simulink model "Copy_of_B747"  (R2022b)
settings: Solver=VariableStepAuto  StartTime=0.0  StopTime=Inf  RelTol=1e-3
undefined symbols (not defined in the file): Initial_cond, Interpolation, out_tr
libraries: simulink_extras x9, slpidlib x5, simulink x3, aerolibanimutils x1
settings Model: Creator=Usuario  LastModifiedBy=Usuario

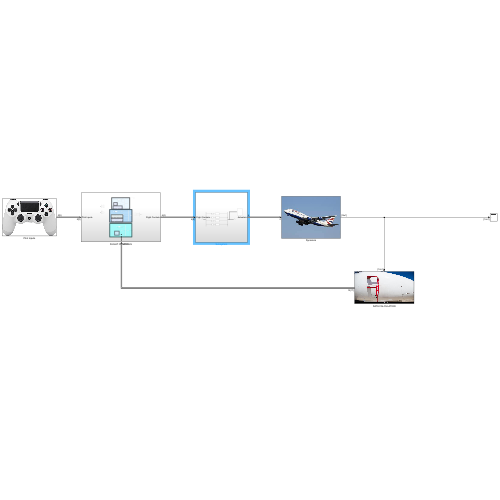
[thumbnail: Simulink's stored preview of the top-level diagram]
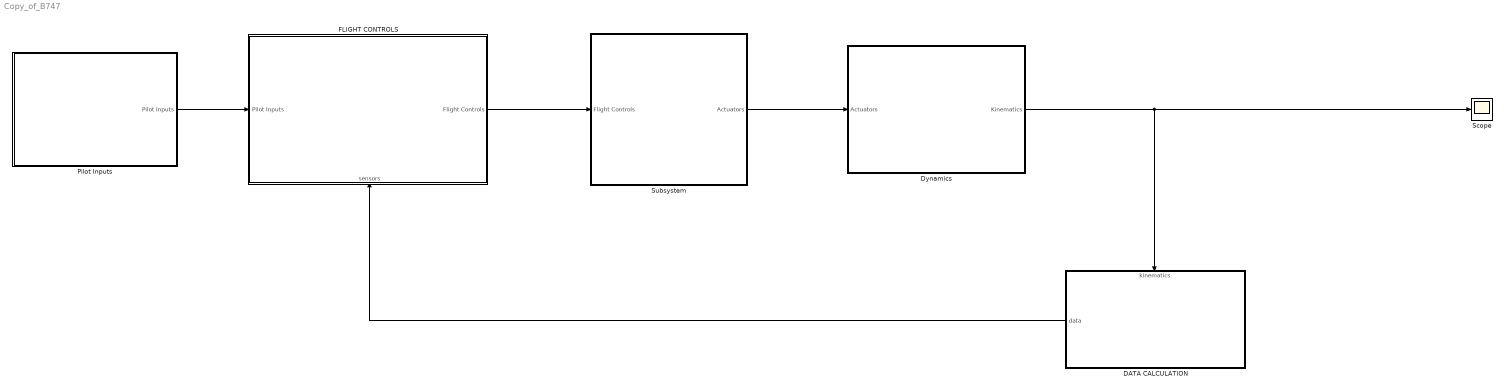
== system Copy_of_B747 ==
  DATA CALCULATION : Subsystem
      settings: PortSchema="{\"entries\":[{\"content\":{\"sides\":[{\"content\":{\"connectorIds\":[\"Out1\"]},\"type\":\"ConnectorPlacement.EquallySpacedRectSide\",\"uuid\":\"3684fda8-23e5-43c4-a1a0-31248e0867f7\"},{\"content\":{\"connectorIds\":[],\"side\":\"RIGHT\"},\"type\":\"ConnectorPlacement.EquallySpacedRectSide\",\"uuid\":\"596d4b37-a63d-424d-8484-dfaf2b397c2c\"},{\"content\":{\"connectorIds\":[\"In1\"],\"side\":\"TOP\"},\"type\":\"ConnectorPlacement.EquallySpacedRectSide\",\"uuid\":\"a12e15c3-f725-45e6-985f-961936170549\"}]},\"type\":\"ConnectorPlacement.EquallySpacedConnector\",\"uuid\":\"9a86d170-49a6-41d6-b658-373aeeb8993b\"}],\"packageUris\":[\"http://schema.mathworks.com/mf0/Connector/R2020b\"],\"version\":\"1.0\"}"
      mask Display: image('C:\Users\Usuario\Documents\MATLAB\B737_simulator\TFM_pics\tubo pitot.jpg'); % Use "Edit Image" on toolstrip to change.
  Dynamics : Subsystem
      mask Display: image('C:\Users\Usuario\Documents\MATLAB\B737_simulator\TFM_pics\b747.jpg'); % Use "Edit Image" on toolstrip to change.
  FLIGHT CONTROLS : Subsystem
      settings: PortSchema="{\"entries\":[{\"content\":{\"sides\":[{\"content\":{\"connectorIds\":[\"In1\"]},\"type\":\"ConnectorPlacement.EquallySpacedRectSide\",\"uuid\":\"91b83ee8-c6ec-4ad7-b4f3-f14dc1cf5d1a\"},{\"content\":{\"connectorIds\":[\"Out1\"],\"side\":\"RIGHT\"},\"type\":\"ConnectorPlacement.EquallySpacedRectSide\",\"uuid\":\"e219be01-4a6e-4062-b72b-ec1396091ca7\"},{\"content\":{\"connectorIds\":[],\"side\":\"TOP\"},\"type\":\"ConnectorPlacement.EquallySpacedRectSide\",\"uuid\":\"96cbe711-5ed8-4304-ab27-a44b299b9c71\"},{\"content\":{\"connectorIds\":[\"In2\"],\"side\":\"BOTTOM\"},\"type\":\"ConnectorPlacement.EquallySpacedRectSide\",\"uuid\":\"b42a0dac-2e5b-48eb-828b-7619874c0cc5\"}]},\"type\":\"ConnectorPlacement.EquallySpacedConnector\",\"uuid\":\"6f7a40d1-3b47-47bb-8706-2539ab3d82b8\"}],\"packageUris\":[\"http://schema.mathworks.com/mf0/Connector/R2020b\"],\"version\":\"1.0\"}"
  Pilot Inputs : Subsystem
      mask Display: image('C:\Users\Usuario\Desktop\mando.jpg'); % Use "Edit Image" on toolstrip to change.
  Scope : Scope
  Subsystem : Subsystem
  wires:
  Dynamics/1(Kinematics) -> Scope/1, DATA CALCULATION/1(kinematics)
  FLIGHT CONTROLS/1(Flight Controls) -> Subsystem/1(Flight Controls)
  DATA CALCULATION/1(data) -> FLIGHT CONTROLS/2(sensors)
  Pilot Inputs/1(Pilot Inputs) -> FLIGHT CONTROLS/1(Pilot Inputs)
  Subsystem/1(Actuators) -> Dynamics/1(Actuators)

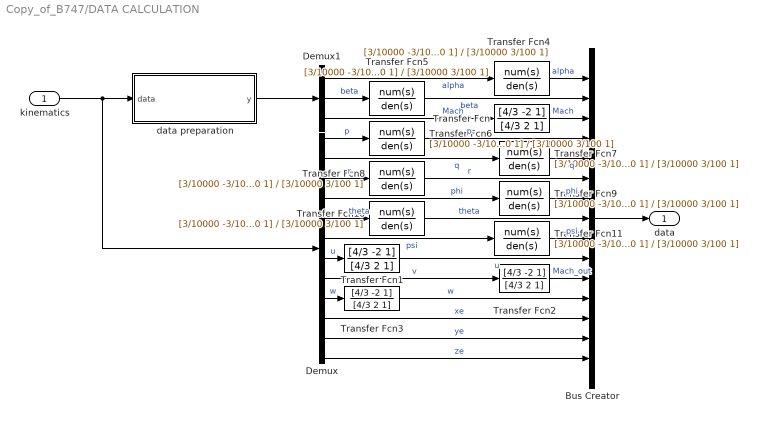
== system Copy_of_B747/DATA CALCULATION ==
  kinematics : Inport
  Bus Creator : BusCreator  Inputs=15
  Demux : Demux  Outputs=12
  Demux1 : Demux  Outputs=3
  Transfer Fcn{,1..3} (4 alike) : TransferFcn  Numerator=[4/3 -2 1]  Denominator=[4/3 2 1]
  Transfer Fcn{4..11} (8 alike) : TransferFcn  Numerator=[3/10000 -3/100 1]  Denominator=[3/10000 3/100 1]
  data preparation : MATLAB Function  TreatAsAtomicUnit=on
  data : Outport
  wires:
  kinematics/1 -> data preparation/1(data), Demux/1
  data preparation/1(y) -> Demux1/1
  Demux1/1 -> Transfer Fcn4/1  "alpha"
  Demux1/2 -> Transfer Fcn5/1  "beta"
  Demux1/3 -> Transfer Fcn/1  "Mach"
  Demux/1 -> Transfer Fcn6/1  "p"
  Demux/2 -> Transfer Fcn7/1  "q"
  Demux/3 -> Transfer Fcn8/1  "r"
  Demux/4 -> Transfer Fcn9/1  "phi"
  Demux/5 -> Transfer Fcn10/1  "theta"
  Demux/6 -> Transfer Fcn11/1  "psi"
  Demux/7 -> Transfer Fcn1/1  "u"
  Demux/8 -> Transfer Fcn2/1  "v"
  Demux/9 -> Transfer Fcn3/1  "w"
  Demux/10 -> Bus Creator/13  "xe"
  Demux/11 -> Bus Creator/14  "ye"
  Demux/12 -> Bus Creator/15  "ze"
  Bus Creator/1 -> data/1
  Transfer Fcn/1 -> Bus Creator/3  "Mach"
  Transfer Fcn1/1 -> Bus Creator/10  "u"
  Transfer Fcn2/1 -> Bus Creator/11  "Mach_out"
  Transfer Fcn3/1 -> Bus Creator/12  "w"
  Transfer Fcn4/1 -> Bus Creator/1  "alpha"
  Transfer Fcn5/1 -> Bus Creator/2  "beta"
  Transfer Fcn6/1 -> Bus Creator/4  "p"
  Transfer Fcn7/1 -> Bus Creator/5  "q"
  Transfer Fcn8/1 -> Bus Creator/6  "r"
  Transfer Fcn9/1 -> Bus Creator/7  "phi"
  Transfer Fcn10/1 -> Bus Creator/8  "theta"
  Transfer Fcn11/1 -> Bus Creator/9  "psi"

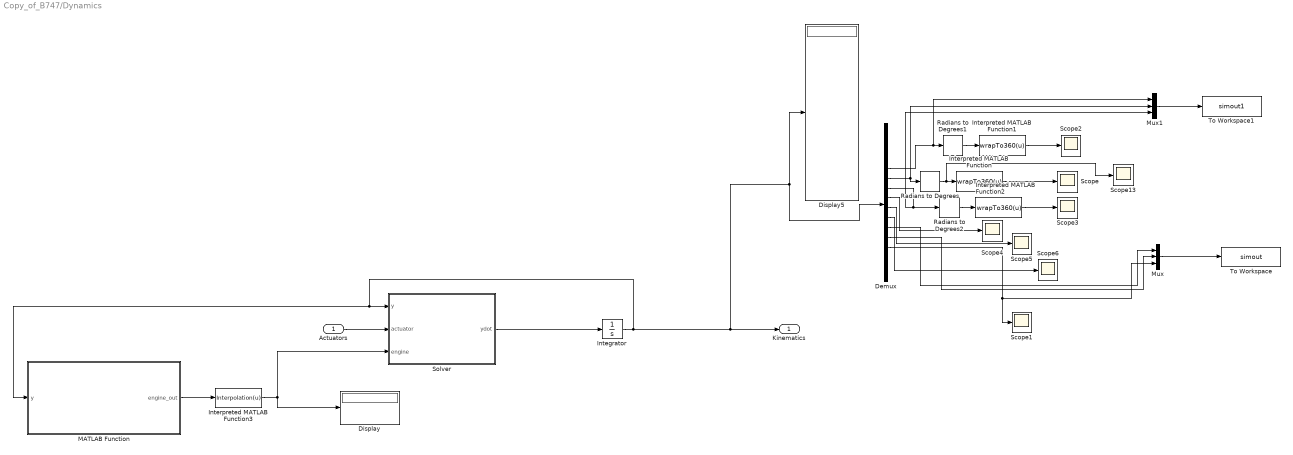
== system Copy_of_B747/Dynamics ==
  Actuators : Inport
  Demux : Demux  Outputs=14
  Display : Display
  Display5 : Display
  Integrator : Integrator  InitialCondition=Initial_cond  ContinuousStateAttributes={'p','q','r','phi','theta','psi','u','v','w','x','y','z','lat','lon'}
  Interpreted MATLAB Function : MATLABFcn  MATLABFcn=wrapTo360(u)
  Interpreted MATLAB Function1 : MATLABFcn  MATLABFcn=wrapTo360(u)
  Interpreted MATLAB Function2 : MATLABFcn  MATLABFcn=wrapTo360(u)
  Interpreted MATLAB Function3 : MATLABFcn  MATLABFcn=Interpolation(u)
  MATLAB Function : MATLAB Function  TreatAsAtomicUnit=on
  Mux : Mux  Inputs=3
  Mux1 : Mux  Inputs=3
  Radians to Degrees : simulink_extras/Transformations/Radians to Degrees
  Radians to Degrees1 : simulink_extras/Transformations/Radians to Degrees
  Radians to Degrees2 : simulink_extras/Transformations/Radians to Degrees
  Scope{,1..6,13} (8 alike) : Scope
  Solver : MATLAB Function  TreatAsAtomicUnit=on
  To Workspace : ToWorkspace  VariableName=simout  SampleTime=-1
  To Workspace1 : ToWorkspace  VariableName=simout1  SampleTime=-1
  Kinematics : Outport
  wires:
  Solver/1(ydot) -> Integrator/1
  Actuators/1 -> Solver/2(actuator)
  Interpreted MATLAB Function3/1 -> Display/1, Solver/3(engine)
  MATLAB Function/1(engine_out) -> Interpreted MATLAB Function3/1
  Demux/11 -> Mux/2
  Mux1/1 -> To Workspace1/1
  Demux/9 -> Scope6/1
  Interpreted MATLAB Function1/1 -> Scope2/1
  Demux/10 -> Mux/1
  Demux/12 -> Scope1/1, Mux/3
  Interpreted MATLAB Function2/1 -> Scope3/1
  Demux/4 -> Mux1/1, Radians to Degrees1/1
  Demux/8 -> Scope5/1
  Demux/6 -> Radians to Degrees2/1, Mux1/3
  Radians to Degrees2/1 -> Interpreted MATLAB Function2/1
  Demux/5 -> Radians to Degrees/1, Mux1/2
  Interpreted MATLAB Function/1 -> Scope/1
  Demux/7 -> Scope4/1
  Radians to Degrees1/1 -> Interpreted MATLAB Function1/1
  Radians to Degrees/1 -> Scope13/1, Interpreted MATLAB Function/1
  Mux/1 -> To Workspace/1
  Integrator/1 -> Solver/1(y), MATLAB Function/1(y), Demux/1, Display5/1, Kinematics/1

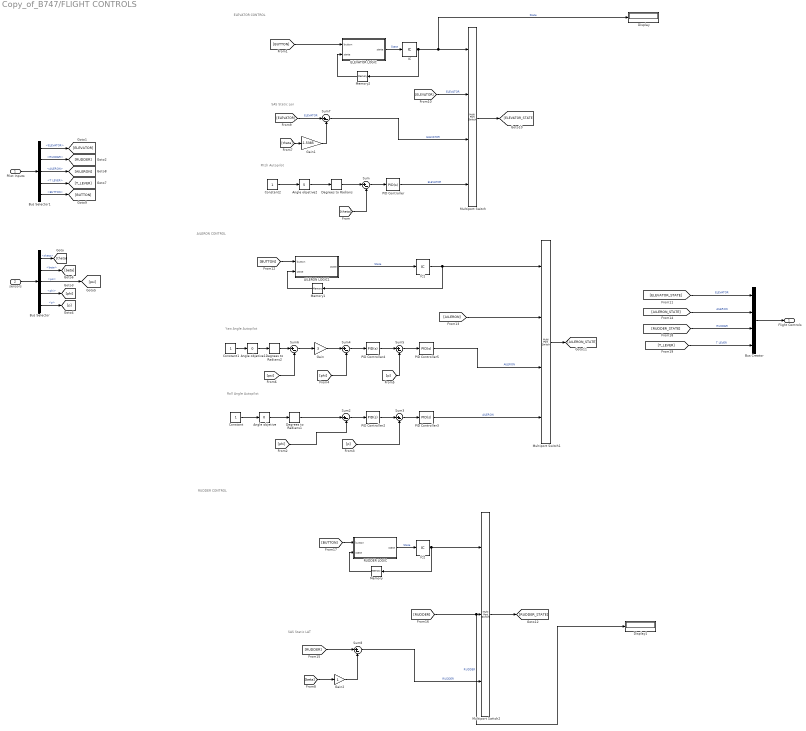
== system Copy_of_B747/FLIGHT CONTROLS ==
  note: RUDDER CONTROL
  note: AILERON CONTROL
  note: ELEVATOR CONTROL
  note: SAS Static LAT
  note: SAS Static Lon
  note: Roll Angle Autopilot
  note: Pitch Autopilot
  note: Yaw Angle Autopilot
  Pilot Inputs : Inport
  sensors : Inport  Port=2
  AILERON LOGIC1 : MATLAB Function  TreatAsAtomicUnit=on
  Angle objetive : simulink/Math Operations/Slider Gain  gain=0  low=-90  high=90
  Angle objetive1 : simulink/Math Operations/Slider Gain  gain=0  low=-180  high=180
  Angle objetive2 : simulink/Math Operations/Slider Gain  gain=5  low=-20  high=20
  Bus Creator : BusCreator  Inputs=4
  Bus Selector : BusSelector  OutputSignals=theta,beta,psi,phi,p
  Bus Selector1 : BusSelector  OutputSignals=ELEVATOR,RUDDER,AILERON,T LEVER,BUTTON
  Constant : Constant
  Constant1 : Constant
  Constant2 : Constant
  Degrees to Radians : simulink_extras/Transformations/Degrees to Radians
  Degrees to Radians1 : simulink_extras/Transformations/Degrees to Radians
  Degrees to Radians2 : simulink_extras/Transformations/Degrees to Radians
  Display : Display
  Display1 : Display
  ELEVATOR LOGIC : MATLAB Function  TreatAsAtomicUnit=on
  Gain : Gain  Gain=3
  Gain1 : Gain  Gain=-1.5385
  Gain2 : Gain
  IC : InitialCondition  Value=3
  IC1 : InitialCondition
  IC2 : InitialCondition
  Memory : Memory
  Memory1 : Memory
  Memory2 : Memory
  Multiport Switch : MultiPortSwitch  SaturateOnIntegerOverflow=off  InputSameDT=off
  Multiport Switch1 : MultiPortSwitch  SaturateOnIntegerOverflow=off  InputSameDT=off
  Multiport Switch2 : MultiPortSwitch  Inputs=2  SaturateOnIntegerOverflow=off  InputSameDT=off
  PID Controller : slpidlib/PID Controller  Controller=PID  Form=Parallel  TimeDomain=Continuous-time  UseExternalTs=off  SampleTime=-1  IntegratorMethod=Forward Euler  FilterMethod=Forward Euler  ControllerParametersSource=internal  P=-0.15  I=-0.05  UseKiTs=off  D=0  N=100  UseFilter=on  TunerSelectOption=Transfer Function Based (PID Tuner App)  InitialConditionSource=internal  InitialConditionForIntegrator=0  InitialConditionForFilter=0  DifferentiatorICPrevScaledInput=0  ExternalReset=none  TrackingMode=off  Kt=1  LimitOutput=off  SatLimitsSource=internal  UpperSaturationLimit=inf  LowerSaturationLimit=-inf  LinearizeAsGain=on  AntiWindupMode=none  Kb=1  LimitIntegrator=off  UpperIntegratorSaturationLimit=inf  LowerIntegratorSaturationLimit=-inf  POutMin=[]  POutMax=[]  IOutMin=[]  IOutMax=[]  DOutMin=[]  DOutMax=[]  NOutMin=[]  NOutMax=[]  SumOutMin=[]  SumOutMax=[]  SaturationOutMin=[]  SaturationOutMax=[]  PParamMin=[]  PParamMax=[]  IParamMin=[]  IParamMax=[]  DParamMin=[]  DParamMax=[]  NParamMin=[]  NParamMax=[]  KbParamMin=[]  KbParamMax=[]  KtParamMin=[]  KtParamMax=[]  KbOutMin=[]  KbOutMax=[]  KtOutMin=[]  KtOutMax=[]  IntegratorOutMin=[]  IntegratorOutMax=[]  FilterOutMin=[]  FilterOutMax=[]  SumI1OutMin=[]  SumI1OutMax=[]  SumI2OutMin=[]  SumI2OutMax=[]  SumI3OutMin=[]  SumI3OutMax=[]  SumI4OutMin=[]  SumI4OutMax=[]  SumDOutMin=[]  SumDOutMax=[]  DifferentiatorOutMin=[]  DifferentiatorOutMax=[]  FilterDiffOutCoefMin=[]  FilterDiffOutCoefMax=[]  ReciprocalOutMin=[]  ReciprocalOutMax=[]  SumDenOutMin=[]  SumDenOutMax=[]  SumNumOutMin=[]  SumNumOutMax=[]  DivideOutMin=[]  DivideOutMax=[]  UdiffTsProdOutMin=[]  UdiffTsProdOutMax=[]  NTsProdOutMin=[]  NTsProdOutMax=[]  UintegralTsProdOutMin=[]  UintegralTsProdOutMax=[]  UngainTsProdOutMin=[]  UngainTsProdOutMax=[]  ClampingZeroOutDataTypeStr=Inherit: Inherit via back propagation  ClampingZeroOutMin=[]  ClampingZeroOutMax=[]  FilterDenConstantOutDataTypeStr=Inherit: Inherit via back propagation  FilterDenConstantOutMin=[]  FilterDenConstantOutMax=[]  PCopyOutDataTypeStr=Inherit: Inherit via back propagation  PCopyOutMin=[]  PCopyOutMax=[]  NCopyOutDataTypeStr=Inherit: Inherit via back propagation  NCopyOutMin=[]  NCopyOutMax=[]  IntegratorContinuousStateAttributes=''  IntegratorStateMustResolveToSignalObject=off  IntegratorRTWStateStorageClass=Auto  FilterContinuousStateAttributes=''  FilterStateMustResolveToSignalObject=off  FilterRTWStateStorageClass=Auto  ParallelPVariant=InternalParameters  IdealPVariant=Disabled  IVariant=InternalParameters  DVariant=InternalParameters  IntegratorVariant=Continuous  SatVariant=Disabled  AWVariant=Passthrough  PCopyVariant=Disabled  TRVariant=Disabled  FdbkBlocksVariant=Forward  IdealPFdbkVariant=Disabled  SatFdbkVariant=Disabled  DerivativeFilterVariant=ContFilter  NVariant=InternalParameters  NCopyVariant=Disabled  FilterICVariant=InternalICsFilter  IntegratorICVariant=InternalICs  ExternalResetVariant=Disabled  TRSumVariant=Passthrough  SumFdbkVariant=Disabled  SumVariant=Sum_PID  TsampFilterVariant=InternalTs  TsampNgainVariant=Passthrough  TsampIntegralVariant=Passthrough  ExternalSaturationOutDataTypeStr=Inherit: Same as second input
  PID Controller2 : slpidlib/PID Controller  Controller=PID  Form=Parallel  TimeDomain=Continuous-time  UseExternalTs=off  SampleTime=-1  IntegratorMethod=Forward Euler  FilterMethod=Forward Euler  ControllerParametersSource=internal  P=0.7  I=0.008  UseKiTs=off  D=0.1  N=100  UseFilter=on  TunerSelectOption=Transfer Function Based (PID Tuner App)  InitialConditionSource=internal  InitialConditionForIntegrator=0  InitialConditionForFilter=0  DifferentiatorICPrevScaledInput=0  ExternalReset=none  TrackingMode=off  Kt=1  LimitOutput=off  SatLimitsSource=internal  UpperSaturationLimit=inf  LowerSaturationLimit=-inf  LinearizeAsGain=on  AntiWindupMode=none  Kb=1  LimitIntegrator=off  UpperIntegratorSaturationLimit=inf  LowerIntegratorSaturationLimit=-inf  POutMin=[]  POutMax=[]  IOutMin=[]  IOutMax=[]  DOutMin=[]  DOutMax=[]  NOutMin=[]  NOutMax=[]  SumOutMin=[]  SumOutMax=[]  SaturationOutMin=[]  SaturationOutMax=[]  PParamMin=[]  PParamMax=[]  IParamMin=[]  IParamMax=[]  DParamMin=[]  DParamMax=[]  NParamMin=[]  NParamMax=[]  KbParamMin=[]  KbParamMax=[]  KtParamMin=[]  KtParamMax=[]  KbOutMin=[]  KbOutMax=[]  KtOutMin=[]  KtOutMax=[]  IntegratorOutMin=[]  IntegratorOutMax=[]  FilterOutMin=[]  FilterOutMax=[]  SumI1OutMin=[]  SumI1OutMax=[]  SumI2OutMin=[]  SumI2OutMax=[]  SumI3OutMin=[]  SumI3OutMax=[]  SumI4OutMin=[]  SumI4OutMax=[]  SumDOutMin=[]  SumDOutMax=[]  DifferentiatorOutMin=[]  DifferentiatorOutMax=[]  FilterDiffOutCoefMin=[]  FilterDiffOutCoefMax=[]  ReciprocalOutMin=[]  ReciprocalOutMax=[]  SumDenOutMin=[]  SumDenOutMax=[]  SumNumOutMin=[]  SumNumOutMax=[]  DivideOutMin=[]  DivideOutMax=[]  UdiffTsProdOutMin=[]  UdiffTsProdOutMax=[]  NTsProdOutMin=[]  NTsProdOutMax=[]  UintegralTsProdOutMin=[]  UintegralTsProdOutMax=[]  UngainTsProdOutMin=[]  UngainTsProdOutMax=[]  ClampingZeroOutDataTypeStr=Inherit: Inherit via back propagation  ClampingZeroOutMin=[]  ClampingZeroOutMax=[]  FilterDenConstantOutDataTypeStr=Inherit: Inherit via back propagation  FilterDenConstantOutMin=[]  FilterDenConstantOutMax=[]  PCopyOutDataTypeStr=Inherit: Inherit via back propagation  PCopyOutMin=[]  PCopyOutMax=[]  NCopyOutDataTypeStr=Inherit: Inherit via back propagation  NCopyOutMin=[]  NCopyOutMax=[]  IntegratorContinuousStateAttributes=''  IntegratorStateMustResolveToSignalObject=off  IntegratorRTWStateStorageClass=Auto  FilterContinuousStateAttributes=''  FilterStateMustResolveToSignalObject=off  FilterRTWStateStorageClass=Auto  ParallelPVariant=InternalParameters  IdealPVariant=Disabled  IVariant=InternalParameters  DVariant=InternalParameters  IntegratorVariant=Continuous  SatVariant=Disabled  AWVariant=Passthrough  PCopyVariant=Disabled  TRVariant=Disabled  FdbkBlocksVariant=Forward  IdealPFdbkVariant=Disabled  SatFdbkVariant=Disabled  DerivativeFilterVariant=ContFilter  NVariant=InternalParameters  NCopyVariant=Disabled  FilterICVariant=InternalICsFilter  IntegratorICVariant=InternalICs  ExternalResetVariant=Disabled  TRSumVariant=Passthrough  SumFdbkVariant=Disabled  SumVariant=Sum_PID  TsampFilterVariant=InternalTs  TsampNgainVariant=Passthrough  TsampIntegralVariant=Passthrough  ExternalSaturationOutDataTypeStr=Inherit: Same as second input
  PID Controller3 : slpidlib/PID Controller  Controller=PID  Form=Parallel  TimeDomain=Continuous-time  UseExternalTs=off  SampleTime=-1  IntegratorMethod=Forward Euler  FilterMethod=Forward Euler  ControllerParametersSource=internal  P=0.4  I=0  UseKiTs=off  D=0  N=100  UseFilter=on  TunerSelectOption=Transfer Function Based (PID Tuner App)  InitialConditionSource=internal  InitialConditionForIntegrator=0  InitialConditionForFilter=0  DifferentiatorICPrevScaledInput=0  ExternalReset=none  TrackingMode=off  Kt=1  LimitOutput=off  SatLimitsSource=internal  UpperSaturationLimit=inf  LowerSaturationLimit=-inf  LinearizeAsGain=on  AntiWindupMode=none  Kb=1  LimitIntegrator=off  UpperIntegratorSaturationLimit=inf  LowerIntegratorSaturationLimit=-inf  POutMin=[]  POutMax=[]  IOutMin=[]  IOutMax=[]  DOutMin=[]  DOutMax=[]  NOutMin=[]  NOutMax=[]  SumOutMin=[]  SumOutMax=[]  SaturationOutMin=[]  SaturationOutMax=[]  PParamMin=[]  PParamMax=[]  IParamMin=[]  IParamMax=[]  DParamMin=[]  DParamMax=[]  NParamMin=[]  NParamMax=[]  KbParamMin=[]  KbParamMax=[]  KtParamMin=[]  KtParamMax=[]  KbOutMin=[]  KbOutMax=[]  KtOutMin=[]  KtOutMax=[]  IntegratorOutMin=[]  IntegratorOutMax=[]  FilterOutMin=[]  FilterOutMax=[]  SumI1OutMin=[]  SumI1OutMax=[]  SumI2OutMin=[]  SumI2OutMax=[]  SumI3OutMin=[]  SumI3OutMax=[]  SumI4OutMin=[]  SumI4OutMax=[]  SumDOutMin=[]  SumDOutMax=[]  DifferentiatorOutMin=[]  DifferentiatorOutMax=[]  FilterDiffOutCoefMin=[]  FilterDiffOutCoefMax=[]  ReciprocalOutMin=[]  ReciprocalOutMax=[]  SumDenOutMin=[]  SumDenOutMax=[]  SumNumOutMin=[]  SumNumOutMax=[]  DivideOutMin=[]  DivideOutMax=[]  UdiffTsProdOutMin=[]  UdiffTsProdOutMax=[]  NTsProdOutMin=[]  NTsProdOutMax=[]  UintegralTsProdOutMin=[]  UintegralTsProdOutMax=[]  UngainTsProdOutMin=[]  UngainTsProdOutMax=[]  ClampingZeroOutDataTypeStr=Inherit: Inherit via back propagation  ClampingZeroOutMin=[]  ClampingZeroOutMax=[]  FilterDenConstantOutDataTypeStr=Inherit: Inherit via back propagation  FilterDenConstantOutMin=[]  FilterDenConstantOutMax=[]  PCopyOutDataTypeStr=Inherit: Inherit via back propagation  PCopyOutMin=[]  PCopyOutMax=[]  NCopyOutDataTypeStr=Inherit: Inherit via back propagation  NCopyOutMin=[]  NCopyOutMax=[]  IntegratorContinuousStateAttributes=''  IntegratorStateMustResolveToSignalObject=off  IntegratorRTWStateStorageClass=Auto  FilterContinuousStateAttributes=''  FilterStateMustResolveToSignalObject=off  FilterRTWStateStorageClass=Auto  ParallelPVariant=InternalParameters  IdealPVariant=Disabled  IVariant=InternalParameters  DVariant=InternalParameters  IntegratorVariant=Continuous  SatVariant=Disabled  AWVariant=Passthrough  PCopyVariant=Disabled  TRVariant=Disabled  FdbkBlocksVariant=Forward  IdealPFdbkVariant=Disabled  SatFdbkVariant=Disabled  DerivativeFilterVariant=ContFilter  NVariant=InternalParameters  NCopyVariant=Disabled  FilterICVariant=InternalICsFilter  IntegratorICVariant=InternalICs  ExternalResetVariant=Disabled  TRSumVariant=Passthrough  SumFdbkVariant=Disabled  SumVariant=Sum_PID  TsampFilterVariant=InternalTs  TsampNgainVariant=Passthrough  TsampIntegralVariant=Passthrough  ExternalSaturationOutDataTypeStr=Inherit: Same as second input
  PID Controller4 : slpidlib/PID Controller  Controller=PID  Form=Parallel  TimeDomain=Continuous-time  UseExternalTs=off  SampleTime=-1  IntegratorMethod=Forward Euler  FilterMethod=Forward Euler  ControllerParametersSource=internal  P=0.7  I=0  UseKiTs=off  D=0  N=100  UseFilter=on  TunerSelectOption=Transfer Function Based (PID Tuner App)  InitialConditionSource=internal  InitialConditionForIntegrator=0  InitialConditionForFilter=0  DifferentiatorICPrevScaledInput=0  ExternalReset=none  TrackingMode=off  Kt=1  LimitOutput=off  SatLimitsSource=internal  UpperSaturationLimit=inf  LowerSaturationLimit=-inf  LinearizeAsGain=on  AntiWindupMode=none  Kb=1  LimitIntegrator=off  UpperIntegratorSaturationLimit=inf  LowerIntegratorSaturationLimit=-inf  POutMin=[]  POutMax=[]  IOutMin=[]  IOutMax=[]  DOutMin=[]  DOutMax=[]  NOutMin=[]  NOutMax=[]  SumOutMin=[]  SumOutMax=[]  SaturationOutMin=[]  SaturationOutMax=[]  PParamMin=[]  PParamMax=[]  IParamMin=[]  IParamMax=[]  DParamMin=[]  DParamMax=[]  NParamMin=[]  NParamMax=[]  KbParamMin=[]  KbParamMax=[]  KtParamMin=[]  KtParamMax=[]  KbOutMin=[]  KbOutMax=[]  KtOutMin=[]  KtOutMax=[]  IntegratorOutMin=[]  IntegratorOutMax=[]  FilterOutMin=[]  FilterOutMax=[]  SumI1OutMin=[]  SumI1OutMax=[]  SumI2OutMin=[]  SumI2OutMax=[]  SumI3OutMin=[]  SumI3OutMax=[]  SumI4OutMin=[]  SumI4OutMax=[]  SumDOutMin=[]  SumDOutMax=[]  DifferentiatorOutMin=[]  DifferentiatorOutMax=[]  FilterDiffOutCoefMin=[]  FilterDiffOutCoefMax=[]  ReciprocalOutMin=[]  ReciprocalOutMax=[]  SumDenOutMin=[]  SumDenOutMax=[]  SumNumOutMin=[]  SumNumOutMax=[]  DivideOutMin=[]  DivideOutMax=[]  UdiffTsProdOutMin=[]  UdiffTsProdOutMax=[]  NTsProdOutMin=[]  NTsProdOutMax=[]  UintegralTsProdOutMin=[]  UintegralTsProdOutMax=[]  UngainTsProdOutMin=[]  UngainTsProdOutMax=[]  ClampingZeroOutDataTypeStr=Inherit: Inherit via back propagation  ClampingZeroOutMin=[]  ClampingZeroOutMax=[]  FilterDenConstantOutDataTypeStr=Inherit: Inherit via back propagation  FilterDenConstantOutMin=[]  FilterDenConstantOutMax=[]  PCopyOutDataTypeStr=Inherit: Inherit via back propagation  PCopyOutMin=[]  PCopyOutMax=[]  NCopyOutDataTypeStr=Inherit: Inherit via back propagation  NCopyOutMin=[]  NCopyOutMax=[]  IntegratorContinuousStateAttributes=''  IntegratorStateMustResolveToSignalObject=off  IntegratorRTWStateStorageClass=Auto  FilterContinuousStateAttributes=''  FilterStateMustResolveToSignalObject=off  FilterRTWStateStorageClass=Auto  ParallelPVariant=InternalParameters  IdealPVariant=Disabled  IVariant=InternalParameters  DVariant=InternalParameters  IntegratorVariant=Continuous  SatVariant=Disabled  AWVariant=Passthrough  PCopyVariant=Disabled  TRVariant=Disabled  FdbkBlocksVariant=Forward  IdealPFdbkVariant=Disabled  SatFdbkVariant=Disabled  DerivativeFilterVariant=ContFilter  NVariant=InternalParameters  NCopyVariant=Disabled  FilterICVariant=InternalICsFilter  IntegratorICVariant=InternalICs  ExternalResetVariant=Disabled  TRSumVariant=Passthrough  SumFdbkVariant=Disabled  SumVariant=Sum_PID  TsampFilterVariant=InternalTs  TsampNgainVariant=Passthrough  TsampIntegralVariant=Passthrough  ExternalSaturationOutDataTypeStr=Inherit: Same as second input
  PID Controller5 : slpidlib/PID Controller  Controller=PID  Form=Parallel  TimeDomain=Continuous-time  UseExternalTs=off  SampleTime=-1  IntegratorMethod=Forward Euler  FilterMethod=Forward Euler  ControllerParametersSource=internal  P=0.4  I=0  UseKiTs=off  D=0  N=100  UseFilter=on  TunerSelectOption=Transfer Function Based (PID Tuner App)  InitialConditionSource=internal  InitialConditionForIntegrator=0  InitialConditionForFilter=0  DifferentiatorICPrevScaledInput=0  ExternalReset=none  TrackingMode=off  Kt=1  LimitOutput=off  SatLimitsSource=internal  UpperSaturationLimit=inf  LowerSaturationLimit=-inf  LinearizeAsGain=on  AntiWindupMode=none  Kb=1  LimitIntegrator=off  UpperIntegratorSaturationLimit=inf  LowerIntegratorSaturationLimit=-inf  POutMin=[]  POutMax=[]  IOutMin=[]  IOutMax=[]  DOutMin=[]  DOutMax=[]  NOutMin=[]  NOutMax=[]  SumOutMin=[]  SumOutMax=[]  SaturationOutMin=[]  SaturationOutMax=[]  PParamMin=[]  PParamMax=[]  IParamMin=[]  IParamMax=[]  DParamMin=[]  DParamMax=[]  NParamMin=[]  NParamMax=[]  KbParamMin=[]  KbParamMax=[]  KtParamMin=[]  KtParamMax=[]  KbOutMin=[]  KbOutMax=[]  KtOutMin=[]  KtOutMax=[]  IntegratorOutMin=[]  IntegratorOutMax=[]  FilterOutMin=[]  FilterOutMax=[]  SumI1OutMin=[]  SumI1OutMax=[]  SumI2OutMin=[]  SumI2OutMax=[]  SumI3OutMin=[]  SumI3OutMax=[]  SumI4OutMin=[]  SumI4OutMax=[]  SumDOutMin=[]  SumDOutMax=[]  DifferentiatorOutMin=[]  DifferentiatorOutMax=[]  FilterDiffOutCoefMin=[]  FilterDiffOutCoefMax=[]  ReciprocalOutMin=[]  ReciprocalOutMax=[]  SumDenOutMin=[]  SumDenOutMax=[]  SumNumOutMin=[]  SumNumOutMax=[]  DivideOutMin=[]  DivideOutMax=[]  UdiffTsProdOutMin=[]  UdiffTsProdOutMax=[]  NTsProdOutMin=[]  NTsProdOutMax=[]  UintegralTsProdOutMin=[]  UintegralTsProdOutMax=[]  UngainTsProdOutMin=[]  UngainTsProdOutMax=[]  ClampingZeroOutDataTypeStr=Inherit: Inherit via back propagation  ClampingZeroOutMin=[]  ClampingZeroOutMax=[]  FilterDenConstantOutDataTypeStr=Inherit: Inherit via back propagation  FilterDenConstantOutMin=[]  FilterDenConstantOutMax=[]  PCopyOutDataTypeStr=Inherit: Inherit via back propagation  PCopyOutMin=[]  PCopyOutMax=[]  NCopyOutDataTypeStr=Inherit: Inherit via back propagation  NCopyOutMin=[]  NCopyOutMax=[]  IntegratorContinuousStateAttributes=''  IntegratorStateMustResolveToSignalObject=off  IntegratorRTWStateStorageClass=Auto  FilterContinuousStateAttributes=''  FilterStateMustResolveToSignalObject=off  FilterRTWStateStorageClass=Auto  ParallelPVariant=InternalParameters  IdealPVariant=Disabled  IVariant=InternalParameters  DVariant=InternalParameters  IntegratorVariant=Continuous  SatVariant=Disabled  AWVariant=Passthrough  PCopyVariant=Disabled  TRVariant=Disabled  FdbkBlocksVariant=Forward  IdealPFdbkVariant=Disabled  SatFdbkVariant=Disabled  DerivativeFilterVariant=ContFilter  NVariant=InternalParameters  NCopyVariant=Disabled  FilterICVariant=InternalICsFilter  IntegratorICVariant=InternalICs  ExternalResetVariant=Disabled  TRSumVariant=Passthrough  SumFdbkVariant=Disabled  SumVariant=Sum_PID  TsampFilterVariant=InternalTs  TsampNgainVariant=Passthrough  TsampIntegralVariant=Passthrough  ExternalSaturationOutDataTypeStr=Inherit: Same as second input
  RUDDER LOGIC : MATLAB Function  TreatAsAtomicUnit=on
  Sum{,2..8} (8 alike) : Sum  Inputs=|+-
  Flight Controls : Outport
  wires:
  sensors/1 -> Bus Selector/1
  Bus Selector/1 -> [theta]  "<theta>"
  Degrees to Radians/1 -> Sum/1
  PID Controller/1 -> Multiport Switch/4  "ELEVATOR"
  [theta] -> Sum/2
  Sum/1 -> PID Controller/1
  Bus Selector/3 -> [psi]  "<psi>"
  Bus Selector/2 -> [beta]  "<beta>"
  Angle objetive/1 -> Degrees to Radians1/1
  Sum2/1 -> PID Controller2/1
  Bus Selector/4 -> [phi]  "<phi>"
  Bus Selector/5 -> [p]  "<p>"
  [phi] -> Sum2/2
  PID Controller2/1 -> Sum3/1
  [p] -> Sum3/2
  Sum3/1 -> PID Controller3/1
  PID Controller3/1 -> Multiport Switch1/4  "AILERON"
  Sum5/1 -> PID Controller5/1
  PID Controller5/1 -> Multiport Switch1/3  "AILERON"
  [phi] -> Sum4/2
  PID Controller4/1 -> Sum5/1
  Sum4/1 -> PID Controller4/1
  [p] -> Sum5/2
  Degrees to Radians2/1 -> Sum6/1
  Sum6/1 -> Gain/1
  Gain/1 -> Sum4/1
  [psi] -> Sum6/2
  Sum7/1 -> Multiport Switch/3  "ELEVATOR"
  [ELEVATOR] -> Sum7/1  "ELEVATOR"
  [theta] -> Gain1/1
  Gain1/1 -> Sum7/2
  [RUDDER] -> Sum8/1
  [beta] -> Gain2/1
  Gain2/1 -> Sum8/2
  Sum8/1 -> Multiport Switch2/3  "RUDDER"
  Pilot Inputs/1 -> Bus Selector1/1
  [ELEVATOR_STATE] -> Bus Creator/1  "ELEVATOR"
  [AILERON_STATE] -> Bus Creator/2  "AILERON"
  [RUDDER_STATE] -> Bus Creator/3  "RUDDER"
  [T_LEVER] -> Bus Creator/4  "T LEVER"
  Bus Creator/1 -> Flight Controls/1
  Bus Selector1/1 -> [ELEVATOR]  "<ELEVATOR>"
  Bus Selector1/2 -> [RUDDER]  "<RUDDER>"
  Bus Selector1/3 -> [AILERON]  "<AILERON>"
  Bus Selector1/4 -> [T_LEVER]  "<T LEVER>"
  Bus Selector1/5 -> [BUTTON]  "<BUTTON>"
  [BUTTON] -> ELEVATOR LOGIC/1(button)
  [ELEVATOR] -> Multiport Switch/2  "ELEVATOR"
  Multiport Switch/1 -> [ELEVATOR_STATE]
  [BUTTON] -> AILERON LOGIC1/1(button)
  AILERON LOGIC1/1(state) -> IC1/1  "State"
  [AILERON] -> Multiport Switch1/2
  Multiport Switch1/1 -> [AILERON_STATE]
  [RUDDER] -> Display1/1, Multiport Switch2/2  "RUDDER"
  RUDDER LOGIC/1(state) -> IC2/1  "State"
  [BUTTON] -> RUDDER LOGIC/1(button)
  Multiport Switch2/1 -> [RUDDER_STATE]
  Memory/1 -> RUDDER LOGIC/2("state ")
  Memory1/1 -> AILERON LOGIC1/2("state ")
  Memory2/1 -> ELEVATOR LOGIC/2("state ")
  ELEVATOR LOGIC/1(state) -> IC/1  "State"
  IC1/1 -> Memory1/1, Multiport Switch1/1
  IC2/1 -> Memory/1, Multiport Switch2/1
  Constant/1 -> Angle objetive/1
  Degrees to Radians1/1 -> Sum2/1
  Angle objetive1/1 -> Degrees to Radians2/1
  Constant1/1 -> Angle objetive1/1
  Constant2/1 -> Angle objetive2/1
  Angle objetive2/1 -> Degrees to Radians/1
  IC/1 -> Memory2/1, Display/1, Multiport Switch/1  "State"

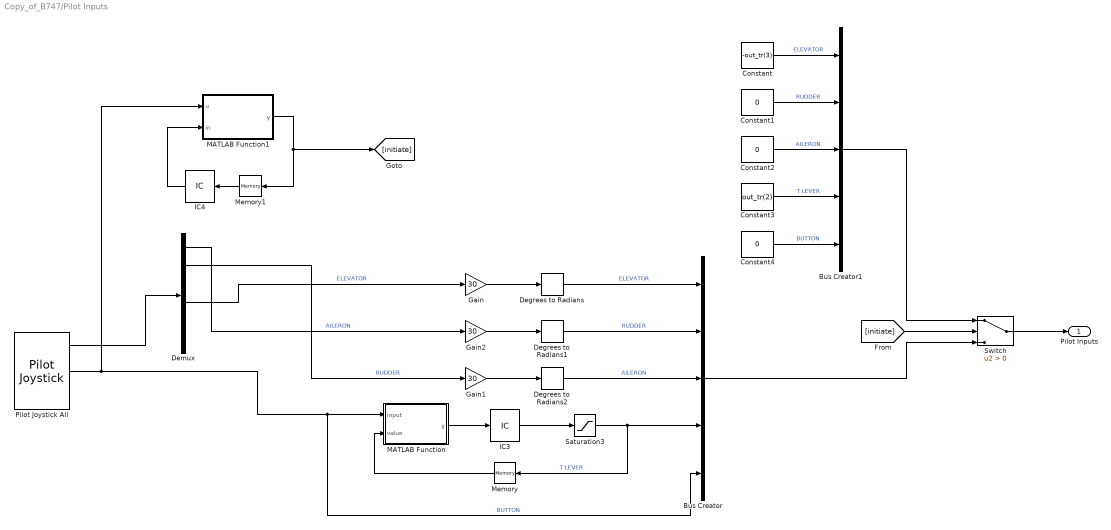
== system Copy_of_B747/Pilot Inputs ==
  Bus Creator : BusCreator  Inputs=5
  Bus Creator1 : BusCreator  Inputs=5
  Constant : Constant  Value=-out_tr(3)
  Constant1 : Constant  Value=0
  Constant2 : Constant  Value=0
  Constant3 : Constant  Value=out_tr(2)
  Constant4 : Constant  Value=0
  Degrees to Radians : simulink_extras/Transformations/Degrees to Radians
  Degrees to Radians1 : simulink_extras/Transformations/Degrees to Radians
  Degrees to Radians2 : simulink_extras/Transformations/Degrees to Radians
  Demux : Demux  Outputs=6
  Gain : Gain  Gain=30
  Gain1 : Gain  Gain=30
  Gain2 : Gain  Gain=30
  IC3 : InitialCondition  Value=out_tr(2)
  IC4 : InitialCondition
  MATLAB Function : MATLAB Function  TreatAsAtomicUnit=on
  MATLAB Function1 : MATLAB Function  TreatAsAtomicUnit=on
  Memory : Memory
  Memory1 : Memory
  Pilot Joystick All : aerolibanimutils/Pilot Joystick  JoystickID=Joystick1  OutputConfiguration=AllOutputs  SampleTime=1/30
      settings: LibrarySourceBlock=aerolibanimutils/Pilot Joystick All
  Saturation3 : Saturate  UpperLimit=1  LowerLimit=0
  Switch : Switch  Criteria=u2 > Threshold  SaturateOnIntegerOverflow=off  InputSameDT=off
  Pilot Inputs : Outport
  wires:
  Bus Creator/1 -> Switch/3
  Gain/1 -> Degrees to Radians/1
  Gain2/1 -> Degrees to Radians1/1
  Gain1/1 -> Degrees to Radians2/1
  Degrees to Radians/1 -> Bus Creator/1  "ELEVATOR"
  Degrees to Radians1/1 -> Bus Creator/2  "RUDDER"
  Degrees to Radians2/1 -> Bus Creator/3  "AILERON"
  Pilot Joystick All/1 -> Demux/1
  Pilot Joystick All/2 -> MATLAB Function1/1(u), Bus Creator/5, MATLAB Function/1(input)  "BUTTON"
  Demux/1 -> Gain2/1  "AILERON"
  Demux/2 -> Gain1/1  "RUDDER"
  Demux/4 -> Gain/1  "ELEVATOR"
  MATLAB Function/1(y) -> IC3/1
  Memory/1 -> MATLAB Function/2(value)
  Saturation3/1 -> Memory/1, Bus Creator/4  "T LEVER"
  IC3/1 -> Saturation3/1
  MATLAB Function1/1(y) -> Memory1/1, [initiate]
  Memory1/1 -> IC4/1
  IC4/1 -> MATLAB Function1/2(in)
  Constant/1 -> Bus Creator1/1  "ELEVATOR"
  Constant1/1 -> Bus Creator1/2  "RUDDER"
  Constant2/1 -> Bus Creator1/3  "AILERON"
  Constant3/1 -> Bus Creator1/4  "T LEVER"
  Constant4/1 -> Bus Creator1/5  "BUTTON"
  Bus Creator1/1 -> Switch/1
  Switch/1 -> Pilot Inputs/1
  [initiate] -> Switch/2

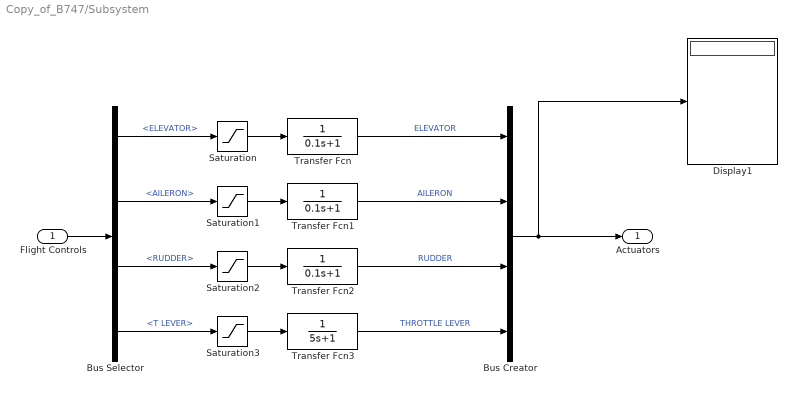
== system Copy_of_B747/Subsystem ==
  Flight Controls : Inport
  Bus Creator : BusCreator  Inputs=4
  Bus Selector : BusSelector  OutputSignals=ELEVATOR,AILERON,RUDDER,T LEVER
  Display1 : Display
  Saturation : Saturate  UpperLimit=30*pi/180  LowerLimit=-30*pi/180
  Saturation1 : Saturate  UpperLimit=30*pi/180  LowerLimit=-30*pi/180
  Saturation2 : Saturate  UpperLimit=30*pi/180  LowerLimit=-30*pi/180
  Saturation3 : Saturate  UpperLimit=1  LowerLimit=0
  Transfer Fcn : TransferFcn  Denominator=[0.1 1]
  Transfer Fcn1 : TransferFcn  Denominator=[0.1 1]
  Transfer Fcn2 : TransferFcn  Denominator=[0.1 1]
  Transfer Fcn3 : TransferFcn  Denominator=[5 1]
  Actuators : Outport
  wires:
  Transfer Fcn2/1 -> Bus Creator/3  "RUDDER"
  Transfer Fcn1/1 -> Bus Creator/2  "AILERON"
  Bus Creator/1 -> Display1/1, Actuators/1
  Transfer Fcn/1 -> Bus Creator/1  "ELEVATOR"
  Transfer Fcn3/1 -> Bus Creator/4  "THROTTLE LEVER"
  Saturation3/1 -> Transfer Fcn3/1
  Saturation2/1 -> Transfer Fcn2/1
  Saturation1/1 -> Transfer Fcn1/1
  Saturation/1 -> Transfer Fcn/1
  Flight Controls/1 -> Bus Selector/1
  Bus Selector/1 -> Saturation/1  "<ELEVATOR>"
  Bus Selector/2 -> Saturation1/1  "<AILERON>"
  Bus Selector/3 -> Saturation2/1  "<RUDDER>"
  Bus Selector/4 -> Saturation3/1  "<T LEVER>"

== matlab function Copy_of_B747/FLIGHT CONTROLS/ELEVATOR LOGIC ==
  data: button input; state output; state input
function state  = elevator_logic(button, state)

if button == 2
    if state == 3
        state = 1;
    else
        state = state + 1;
    end
end

== matlab function Copy_of_B747/Dynamics/Solver ==
  data: y input; actuator input; ydot output; engine input
function ydot  = solver(y,actuator, engine)
%% Definition of constants
g = 9.81;  % acceleration of gravity [m/s^2]
R = 6378137.0; % Earth radius [m]
finv = 298.257222101;
f = 1/finv;
e2 = 1-(1-f)*(1-f);
%% Geometry data
c = 27.3 * 0.3048;
b = 196 * 0.3048;
S = 5500 * (0.3048)^2;
%% Mass properties
% Inertia definition
Ix = 18200000 * 1.3558179619;
Iy = 33100000 * 1.3558179619; 
Iz = 49700000 * 1.3558179619;
Ixz = 11158.75 * 1.3558179619;
% Aircraft mass
m = 636636 * 0.453592; % [kg] -> assumed to be constant

%% Input definition
%% Pilot Inputs
de = actuator(1); % Elevator deflection [rad]
da = actuator(2); % Aileron deflection [rad]
dr = actuator(3); % Rudder deflection [rad]
T_lever = actuator(4); % Throttle lever
%% Definition of variables
%% Angular speeds
p = y(1); % angular speed x-axis [rad/s]
q = y(2); % angular speed y-axis [rad/s]
r = y(3); % angular speed z-axis [rad/s]

%% Euler Angles
phi = y(4); % deg2rad(wrapTo360(rad2deg(y(4)))); % roll angle [rad]
theta =y(5); % deg2rad(wrapTo360(rad2deg(y(5)))); % pitch angle [rad]
psi = y(6); % deg2rad(wrapTo360(rad2deg(y(6)))); % yaw angle [rad]


%% Linear speed
u = y(7); % linear speed x-axis [m/s]
v = y(8); % linear speed y-axis [m/s]
w = y(9); % linear speed z-axis [m/s]

%% Position
xe = y(10); % x-axis earth position
ye = y(11); % y-axis earth position
ze = y(12); % z-axis earth position

%% Latitude and longitude
lambda = wrapTo180(y(13));
long = y(14);

%% Data calculation
V = norm([u,v,w]); % Airspeed [m/s]
alpha = atan2(w,u);
beta = asin(v/V);
atm = atmospheric_model(ze);
qdyn = 0.5 * atm(3) * V^2;

%% Engine Calculation
T = engine(1) * T_lever * 1000;

%% Aerodynamic Forces
%% Aerodynamic Coefficients
%% Longitudinal coefficients
% Drag Coefficients
CD0 = 0.0164; CD_a = 0.2;
% Lift Coefficients
CL0 = 0.21; CL_a = 4.4; Cl_ap = 7.0; CL_q = 6.6; CL_de = 0.32;
% Pitch Coefficients
Cm_0 = 0; Cm_a = -1.0;Cm_ap = -4.0; Cm_q = -20.5; Cm_de = -1.3;

%% Lateral-Directional coefficients
% Side force Coefficients
CY_b = -0.9; CY_p = 0; CY_r = 0.0; CY_da = 0;CY_dr = 0.120;
% Roll Coefficients;
Cl_b = -0.16; Cl_p = -0.34; Cl_r = 0.13; Cl_da = 0.013; Cl_dr = 0.008;
% Yaw Coefficients
Cn_b = 0.16; Cn_p = -0.026; Cn_r = -0.28; Cn_dr = 0.0018; Cn_da = 0.013;

%% Forces calculation
D = qdyn * S * (CD0+CD_a*alpha);
Fy = qdyn * S * (CY_b*beta+CY_p*p*b/(2*V)+CY_r*r*b/(2*V)+CY_da*da+CY_dr*dr);
L = qdyn * S * (CL0+CL_a*alpha+CL_q*q*c/(2*V)+CL_de*de);
Fx = (L*sin(alpha)-D*cos(alpha));
Fz = (-L*cos(alpha)-D*sin(alpha));

%% Torques Calculation
L = qdyn * S * b * (Cl_b*beta+Cl_p*p*b/(2*V)+Cl_r*r*b/(2*V)+Cl_da*da+Cl_dr*dr);
M = qdyn * S * c * (Cm_0+Cm_a*alpha+Cm_q*q*c/(2*V)+Cm_de*de);
N = qdyn * S * b * (Cn_b*beta+Cn_p*p*b/(2*V)+Cn_r*r*b/(2*V)+Cn_dr*dr+Cn_da*da);

%% Equations integration definition
%% Initialization of output vector
ydot = nan(14,1);
    
%% Angular accelerations computation
% x-axix and z-axix obtainded with matlab symbolic math toolbox
ydot(1) = (Iz*L + Ixz*N - Ixz^2*q*r - Iz^2*q*r - Ixz*Iy*p*q +Ixz*Iz*p*q+Ixz*Ix*p*q+ Iy*Iz*q*r)/(Ix*Iz-Ixz^2);

ydot(2) = (M - Ixz*p^2 + Ixz*r^2 - Ix*p*r + Iz*p*r)/Iy;

ydot(3) = (Ixz*L + Ix*N + Ix^2*p*q - Ix*Iy*p*q - Ixz^2*p*q - Ix*Ixz*q*r + Ixz*Iy*q*r - Ixz*Iz*q*r)/(Ix*Iz-Ixz^2);
    
%%  Computation of euler angle rates

ydot(4) = p + (q*sin(phi) + r*cos(phi))*tan(theta);
ydot(5) = q*cos(phi) - r*sin(phi);
ydot(6) = (q*sin(phi) + r*cos(phi))*sec(theta);
    
%% Computation of linear accelerations
% T=0;
ydot(7) = (Fx + T - m*q*w + m*r*v -g*m*sin(theta))/m;
ydot(8) = (Fy + m*p*w - m*r*u + g*m*cos(theta)*sin(phi))/m;
ydot(9) = (Fz - m*p*v + m*q*u + g*m*cos(theta)*cos(phi))/m;

%% Computation of body coordinates

ydot(10) = u*cos(theta)*cos(psi) + v*(sin(phi)*sin(theta)*cos(psi) - cos(phi)*sin(psi))...
    + w*(cos(phi)*sin(theta)*cos(psi) + sin(phi)*sin(psi));
ydot(11) = u*cos(theta)*sin(psi) + v*(sin(phi)*sin(theta)*sin(psi) - cos(phi)*cos(psi))...
    + w*(cos(phi)*sin(theta)*sin(psi) + sin(phi)*cos(psi));
ydot(12) = -(-sin(theta)*u + v*sin(phi)*cos(theta) + w*cos(phi)*cos(theta));

%% Latitude and longitude calculation
v = R./sqrt(1-e2.*sin(lambda)*sin(lambda));
r = v.*(1-e2)./(1-e2*sin(lambda)*sin(lambda));
ydot(13) = xe /(r + ze);
ydot(14) = ye /(cos(lambda)*(R + ze));

%% Output resize matrix
ydot = [ydot(1); ydot(2); ydot(3); ydot(4); ydot(5); ydot(6);...
        ydot(7); ydot(8); ydot(9); ydot(10); ydot(11); ydot(12);...
        ydot(13); ydot(14)];
end

== matlab function Copy_of_B747/Pilot Inputs/MATLAB Function ==
  data: input input; y output; value input
function y = T_lever(input,value)
if input==128
    value = value + 0.01;
elseif input==64
    value = value - 0.01;
end

y = value;

== matlab function Copy_of_B747/DATA CALCULATION/data preparation ==
  data: data input; y output
function y = data_preparation(data)

V = norm([data(7), data(8), data(9)]);
alpha = -atan2(data(9),data(7));
beta = asin(data(8)/V);
atm = atmospheric_model(data(12));
Mach = V / atm(4);

y = [alpha, beta, Mach];

== matlab function Copy_of_B747/FLIGHT CONTROLS/AILERON LOGIC1 ==
  data: button input; state output; state input
function state  = aileron_logic(button, state)

if button == 1
    if state >= 3
        state = 1;
    else
        state = state + 1;
    end
end

== matlab function Copy_of_B747/FLIGHT CONTROLS/RUDDER LOGIC ==
  data: button input; state output; state input
function state  = rudder_logic(button, state)

if button == 8
    if state >= 2
        state = 1;
    else
        state = state + 1;
    end
end

== matlab function Copy_of_B747/Dynamics/MATLAB Function ==
  data: y input; engine_out output
function engine_out = engine_model(y)
%% Function to compute the maximum thrust and fuel flow given altitude and speed
%% Load data from file
% engine = load('engine/Data.mat');
% engine = engine.engine;
%% Initialize output
% engine_out = zeros(1,2);
%% Linear speed
u = y(7); % linear speed x-axis [m/s]
v = y(8); % linear speed y-axis [m/s]
w = y(9); % linear speed z-axis [m/s]

%% Position
ze = y(12); % z-axis earth position

%% Calculate speed norm
tas = sqrt(u^2 + v^2 + w^2);
engine_out = [ze, tas];

% T_interp = scatteredInterpolant(engine(:,1), engine(:,2), engine(:,3));
% ff_interp = scatteredInterpolant(engine(:,1), engine(:,3), engine(:,4));
% 
% engine_out(1) =  T_interp(h,tas);
% engine_out(2) = ff_interp(ze,engine_out(1));

== matlab function Copy_of_B747/Pilot Inputs/MATLAB Function1 ==
  data: u input; y output; in input
function y = initiate_controls(u, in)

if in == 1
    if u == 8192
        in = 0;
    end
end

y = in;
